simulink model "Statechart_Test_All"  (R2016b)
settings: Solver=VariableStepAuto  StartTime=0.0  StopTime=10.0  RelTol=1e-3  EnableMultiTasking=on
settings Model: Creator=Rose  LastModifiedBy=Rose
settings OptimizationCC: DefaultParameterBehavior=Inlined  LifeSpan=inf
settings DebuggingCC: SFUnexpectedBacktrackingDiag=warning  SFNoUnconditionalDefaultTransitionDiag=warning  SFExecutionAtInitializationDiag=none
settings GRTTargetCC: TargetLangStandard=C89/C90 (ANSI)
settings ConfigComp: CovMetricSettings=dw  CovHtmlReporting=on  CovSaveCumulativeToWorkspaceVar=on  CovSaveSingleToWorkspaceVar=on  CovExternalEMLEnable=off

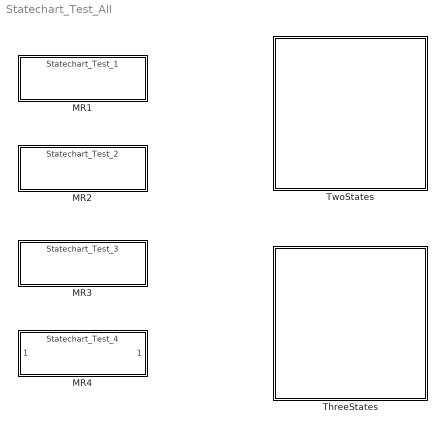
== system Statechart_Test_All ==
  MR1 : ModelReference  ModelNameDialog=Statechart_Test_1  SimulationMode=Normal  ModelReferenceVersion=1.9
  MR2 : ModelReference  ModelNameDialog=Statechart_Test_2  SimulationMode=Normal  ModelReferenceVersion=1.48
  MR3 : ModelReference  ModelNameDialog=Statechart_Test_3  SimulationMode=Normal  ModelReferenceVersion=1.4
  MR4 : ModelReference  ModelNameDialog=Statechart_Test_4  SimulationMode=Normal  ModelReferenceVersion=1.1
  ThreeStates : Stateflow chart  TreatAsAtomicUnit=on
  TwoStates : Stateflow chart  TreatAsAtomicUnit=on

== stateflow chart Statechart_Test_All/ThreeStates ==
  state InitializeSystem
    entry:
    Light = ORANGE;
  state FailState
    entry:
    Light = RED;
  state On
    entry:
    Light = GREEN;
    partsFed = 0;
    during:
    if(any(sensors >= 2))
    partsFed = partsFed + 1;
    end
  (default) -> InitializeSystem
  FailState -> InitializeSystem : [Alarm == 0]
  InitializeSystem -> FailState [order 2] : after(5,sec)
  InitializeSystem -> On [order 1] : [all(sensors>0)]
  On -> FailState : [Alarm ==1]

== stateflow chart Statechart_Test_All/TwoStates ==
  state ON
    entry: y = 1;
  state OFF
    entry: y = -1;
  (default) -> ON
  ON -> OFF : [u<0]
  OFF -> ON : [u>0]
